simulink model "unstable_system_Explicit_MPC"  (R2020a)
settings: configuration reference "unstable_system_config" (kept outside this file)
undefined symbols (not defined in the file): controller_sw
settings Model: DataDictionary=sim_data_unstable_system.sldd  SILPILSystemUnderTest=refmodels  Creator=tshintai  LastModifiedBy=tshintai
settings ConfigSetRef: SourceName=unstable_system_config

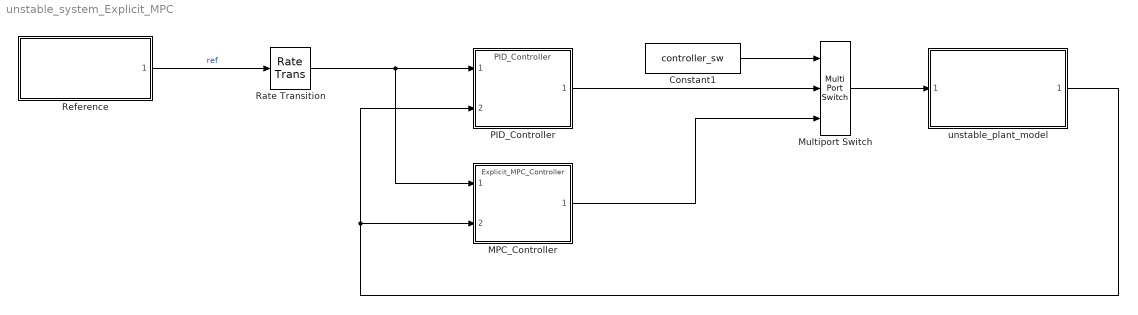
== system unstable_system_Explicit_MPC ==
  Constant1 : Constant  Value=controller_sw  OutDataTypeStr=uint32
  MPC_Controller : ModelReference  ModelNameDialog=Explicit_MPC_Controller  SimulationMode=Normal  ModelReferenceVersion=1.22
  Multiport Switch : MultiPortSwitch  Inputs=2  DiagnosticForDefault=None
  PID_Controller : ModelReference  ModelNameDialog=PID_Controller  SimulationMode=Normal  ModelReferenceVersion=1.81
  Rate Transition : RateTransition  OutPortSampleTime=TimeStep
  Reference : Subsystem  ReferencedSubsystem=Reference_unstable
  unstable_plant_model : Subsystem  ReferencedSubsystem=Unstable_plant_model
  wires:
  Rate Transition/1 -> PID_Controller/1, MPC_Controller/1
  Multiport Switch/1 -> unstable_plant_model/1
  unstable_plant_model/1 -> PID_Controller/2, MPC_Controller/2
  MPC_Controller/1 -> Multiport Switch/3
  Constant1/1 -> Multiport Switch/1
  Reference/1 -> Rate Transition/1  "ref"
  PID_Controller/1 -> Multiport Switch/2
